simulink model "control_model_1D_v2"  (R2025b)
settings: Solver=VariableStepAuto  StartTime=0.0  StopTime=10  RelTol=1e-3
undefined symbols (not defined in the file): engine_gimbal_speed, engine_max_angle, g, gain, initial_position, initial_teta, initial_velocity, Iy, kd, kd_t, kp, kp_t, Kr, Kx, mass, max_thrust, sigma, static_margin
libraries: simulink_extras x4
settings Model: Creator=marti  LastModifiedBy=marti

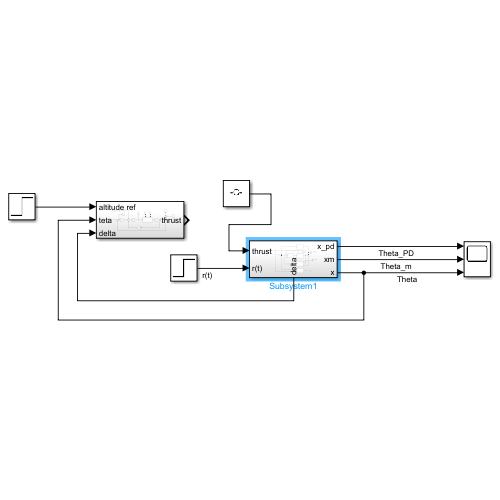
[thumbnail: Simulink's stored preview of the top-level diagram]
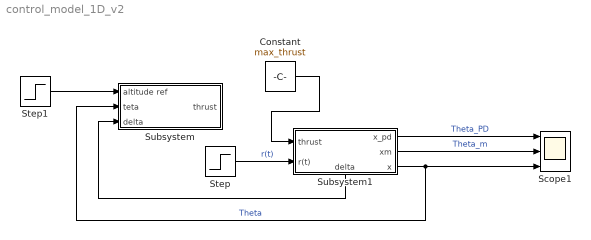
== system control_model_1D_v2 ==
  Constant : Constant  Value=max_thrust
  Scope1 : Scope  NumInputPorts=3
      settings: ActiveDisplayYMinimum=-1.6412064718463906  ActiveDisplayYMaximum=14.77085824661752
  Step : Step  Before=initial_teta  After=10  SampleTime=0
  Step1 : Step  After=30  SampleTime=0
  Subsystem : Subsystem
  Subsystem1 : Subsystem
      settings: PortSchema="{\"entries\":[{\"content\":{\"sides\":[{\"content\":{\"connectorIds\":[\"In1\",\"In2\"]},\"type\":\"ConnectorPlacement.EquallySpacedRectSide\",\"uuid\":\"41c30777-45a1-4158-aee6-2356aa4b2cc5\"},{\"content\":{\"connectorIds\":[\"Out1\",\"Out2\",\"Out3\"],\"side\":\"RIGHT\"},\"type\":\"ConnectorPlacement.EquallySpacedRectSide\",\"uuid\":\"fbc810ba-f647-48d5-9a79-9c3fa84944c8\"},{\"content\":{\"side\":\"TOP\"},\"type\":\"ConnectorPlacement.EquallySpacedRectSide\",\"uuid\":\"5da60fab-04d4-4aae-8ae1-a9a5fc9cdb5d\"},{\"content\":{\"connectorIds\":[\"Out4\"],\"side\":\"BOTTOM\"},\"type\":\"ConnectorPlacement.EquallySpacedRectSide\",\"uuid\":\"fa96aa9e-dc15-4c7b-bdde-b0db6a17889e\"}]},\"type\":\"ConnectorPlacement.EquallySpacedConnector\",\"uuid\":\"2ab61ab6-63dc-40be-af51-040989328b07\"}],\"packageUris\":[\"http://schema.mathworks.com/mf0/Connector/R2020b\"],\"version\":\"1.0\"}"
  wires:
  Step1/1 -> Subsystem/1(altitude ref)
  Step/1 -> Subsystem1/2(r(t))  "r(t)"
  Subsystem1/3(x) -> Subsystem/2(teta), Scope1/3  "Theta"
  Subsystem1/4(delta) -> Subsystem/3(delta)
  Constant/1 -> Subsystem1/1(thrust)
  Subsystem1/2(xm) -> Scope1/2  "Theta_m"
  Subsystem1/1(x_pd) -> Scope1/1  "Theta_PD"

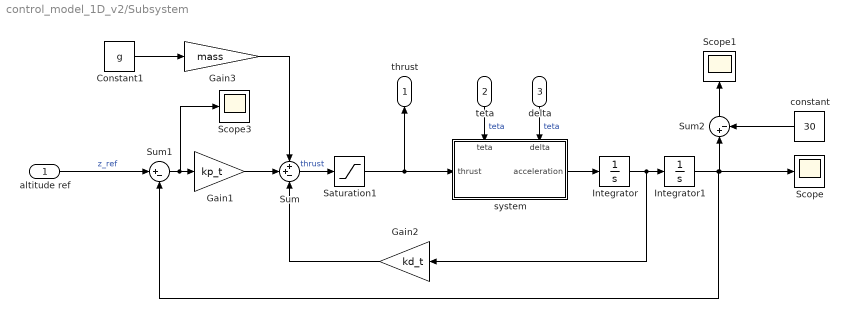
== system control_model_1D_v2/Subsystem ==
  altitude ref : Inport
  teta : Inport  Port=2
  delta : Inport  Port=3
  Constant1 : Constant  Value=g
  Gain1 : Gain  Gain=kp_t
  Gain2 : Gain  Gain=kd_t
  Gain3 : Gain  Gain=mass
  Integrator : Integrator  InitialCondition=initial_velocity
  Integrator1 : Integrator  InitialCondition=initial_position
  Saturation1 : Saturate  UpperLimit=max_thrust  LowerLimit=0
  Scope : Scope
      settings: ActiveDisplayYMinimum=-203.34625268465874  ActiveDisplayYMaximum=578.14958363162873  DataLoggingVariableName=ScopeData7
  Scope1 : Scope
      settings: ActiveDisplayYMinimum=-0.900366360338765  ActiveDisplayYMaximum=1.8353888602601565  DataLoggingVariableName=ScopeData9
  Scope3 : Scope
      settings: ActiveDisplayYMinimum=-1  ActiveDisplayYMaximum=1  DataLoggingVariableName=ScopeData10
  Sum : Sum  Inputs=++-
  Sum1 : Sum  Inputs=|+-
  Sum2 : Sum  Inputs=|+-
  constant : Constant  Value=30
  system : Subsystem
      settings: PortSchema="{\"entries\":[{\"content\":{\"sides\":[{\"content\":{\"connectorIds\":[\"In1\"]},\"type\":\"ConnectorPlacement.EquallySpacedRectSide\",\"uuid\":\"38ff2807-5c3f-4880-9c07-8b6447135695\"},{\"content\":{\"connectorIds\":[\"Out1\"],\"side\":\"RIGHT\"},\"type\":\"ConnectorPlacement.EquallySpacedRectSide\",\"uuid\":\"bc1e5b06-9245-4ba5-abe1-979ca83ec99f\"},{\"content\":{\"connectorIds\":[\"In2\",\"In3\"],\"side\":\"TOP\"},\"type\":\"ConnectorPlacement.EquallySpacedRectSide\",\"uuid\":\"205a83f4-1465-412a-8e3f-6475f5e18be2\"}]},\"type\":\"ConnectorPlacement.EquallySpacedConnector\",\"uuid\":\"dff9f67b-b046-4801-81e2-6dc88e83eb4a\"}],\"packageUris\":[\"http://schema.mathworks.com/mf0/Connector/R2020b\"],\"version\":\"1.0\"}"
  thrust : Outport
  wires:
  system/1(acceleration) -> Integrator/1
  Integrator1/1 -> Scope/1, Sum2/1, Sum1/2
  Gain1/1 -> Sum/2
  Gain2/1 -> Sum/3
  Sum/1 -> Saturation1/1  "thrust"
  Sum1/1 -> Scope3/1, Gain1/1
  Integrator/1 -> Gain2/1, Integrator1/1
  Gain3/1 -> Sum/1
  Constant1/1 -> Gain3/1
  Saturation1/1 -> system/1(thrust), thrust/1
  altitude ref/1 -> Sum1/1  "z_ref"
  teta/1 -> system/2(teta)  "teta"
  constant/1 -> Sum2/2
  Sum2/1 -> Scope1/1
  delta/1 -> system/3(delta)  "teta"

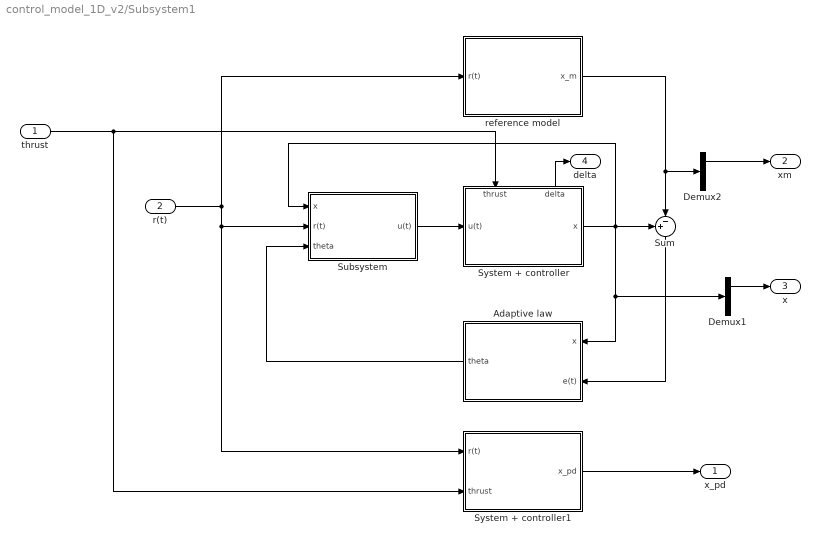
== system control_model_1D_v2/Subsystem1 ==
  thrust : Inport
  r(t) : Inport  Port=2
  Adaptive law : Subsystem  TreatAsAtomicUnit=on
  Demux1 : Demux  Outputs=2
  Demux2 : Demux  Outputs=2
  Subsystem : Subsystem
  Sum : Sum  Inputs=+-|
  System + controller : Subsystem  TreatAsAtomicUnit=on
      settings: PortSchema="{\"entries\":[{\"content\":{\"sides\":[{\"content\":{\"connectorIds\":[\"In1\"]},\"type\":\"ConnectorPlacement.EquallySpacedRectSide\",\"uuid\":\"2888ac6a-c40c-4cbc-ab95-9cb0d58d2b5f\"},{\"content\":{\"connectorIds\":[\"Out1\"],\"side\":\"RIGHT\"},\"type\":\"ConnectorPlacement.EquallySpacedRectSide\",\"uuid\":\"92af2965-0673-45a9-9c50-ea344a811226\"},{\"content\":{\"connectorIds\":[\"In2\",\"Out2\"],\"side\":\"TOP\"},\"type\":\"ConnectorPlacement.EquallySpacedRectSide\",\"uuid\":\"493763d9-5d0c-4185-aada-33137c4c3c69\"}]},\"type\":\"ConnectorPlacement.EquallySpacedConnector\",\"uuid\":\"efbf835c-12ee-4cd9-bf50-b22f4e1c27f3\"}],\"packageUris\":[\"http://schema.mathworks.com/mf0/Connector/R2020b\"],\"version\":\"1.0\"}"
  System + controller1 : Subsystem  TreatAsAtomicUnit=on
  reference model : Subsystem  TreatAsAtomicUnit=on
  x_pd : Outport
  xm : Outport  Port=2
  x : Outport  Port=3
  delta : Outport  Port=4
  wires:
  thrust/1 -> System + controller/2(thrust), System + controller1/2(thrust)
  reference model/1(x_m) -> Demux2/1, Sum/2
  System + controller/1(x) -> Demux1/1, Adaptive law/1(x), Subsystem/1(x), Sum/1
  r(t)/1 -> Subsystem/2(r(t)), System + controller1/1(r(t)), reference model/1(r(t))
  Adaptive law/1(theta) -> Subsystem/3(theta)
  Sum/1 -> Adaptive law/2(e(t))
  System + controller/2(delta) -> delta/1
  System + controller1/1(x_pd) -> x_pd/1
  Demux1/1 -> x/1
  Demux2/1 -> xm/1
  Subsystem/1(u(t)) -> System + controller/1(u(t))

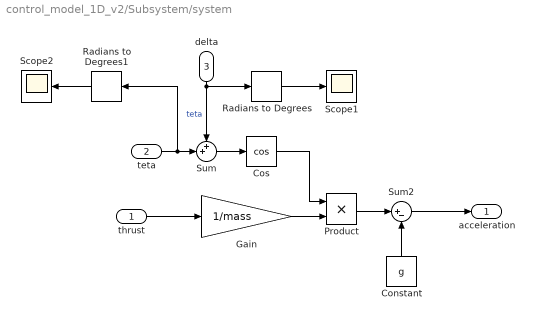
== system control_model_1D_v2/Subsystem/system ==
  thrust : Inport
  teta : Inport  Port=2
  delta : Inport  Port=3
  Constant : Constant  Value=g
  Cos : Trigonometry  Operator=cos
  Gain : Gain  Gain=1/mass
  Product : Product
  Radians to Degrees : simulink_extras/Transformations/Radians to Degrees
  Radians to Degrees1 : simulink_extras/Transformations/Radians to Degrees
  Scope1 : Scope
      settings: ActiveDisplayYMinimum=-1  ActiveDisplayYMaximum=1  DataLoggingVariableName=ScopeData12
  Scope2 : Scope
      settings: ActiveDisplayYMinimum=-1  ActiveDisplayYMaximum=1  DataLoggingVariableName=ScopeData13
  Sum : Sum  Inputs=++|
  Sum2 : Sum  Inputs=|+-
  acceleration : Outport
  wires:
  Constant/1 -> Sum2/2
  Sum2/1 -> acceleration/1
  thrust/1 -> Gain/1
  Gain/1 -> Product/2
  Product/1 -> Sum2/1
  Cos/1 -> Product/1
  teta/1 -> Radians to Degrees1/1, Sum/2
  delta/1 -> Sum/1, Radians to Degrees/1  "teta"
  Sum/1 -> Cos/1
  Radians to Degrees/1 -> Scope1/1
  Radians to Degrees1/1 -> Scope2/1

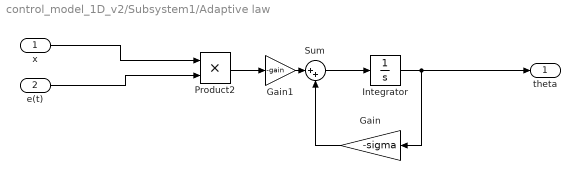
== system control_model_1D_v2/Subsystem1/Adaptive law ==
  x : Inport
  e(t) : Inport  Port=2
  Gain : Gain  Gain=-sigma
  Gain1 : Gain  Gain=-gain
  Integrator : Integrator
  Product2 : Product
  Sum : Sum  Inputs=|++
  theta : Outport
  wires:
  Integrator/1 -> Gain/1, theta/1
  Sum/1 -> Integrator/1
  Gain/1 -> Sum/2
  Gain1/1 -> Sum/1
  Product2/1 -> Gain1/1
  x/1 -> Product2/1
  e(t)/1 -> Product2/2

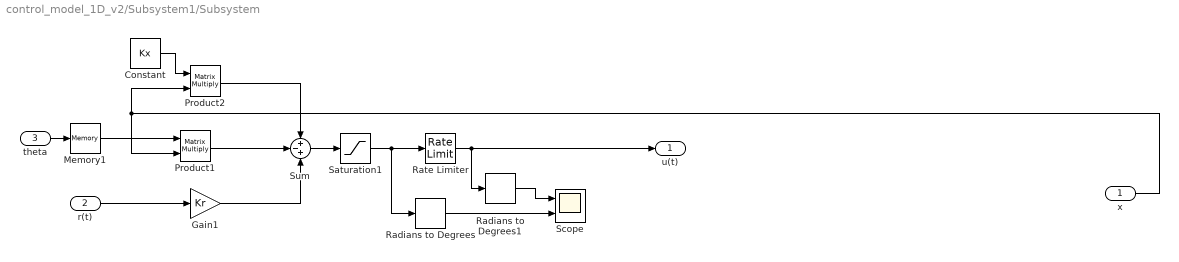
== system control_model_1D_v2/Subsystem1/Subsystem ==
  x : Inport
  r(t) : Inport  Port=2
  theta : Inport  Port=3
  Constant : Constant  Value=Kx  VectorParams1D=off
  Gain1 : Gain  Gain=Kr
  Memory1 : Memory
  Product1 : Product  Multiplication=Matrix(*)
  Product2 : Product  Multiplication=Matrix(*)
  Radians to Degrees : simulink_extras/Transformations/Radians to Degrees
  Radians to Degrees1 : simulink_extras/Transformations/Radians to Degrees
  Rate Limiter : RateLimiter  RisingSlewLimit=engine_gimbal_speed  FallingSlewLimit=-engine_gimbal_speed  SampleTimeMode=inherited
  Saturation1 : Saturate  UpperLimit=engine_max_angle  LowerLimit=-engine_max_angle
  Scope : Scope  NumInputPorts=2
      settings: ActiveDisplayYMinimum=-0.14117420065901104  ActiveDisplayYMaximum=0.22600812143216731
  Sum : Sum  Inputs=+-+
  u(t) : Outport
  wires:
  Radians to Degrees1/1 -> Scope/1
  Memory1/1 -> Product1/1
  r(t)/1 -> Gain1/1
  x/1 -> Product2/2, Product1/2
  Product2/1 -> Sum/1
  Saturation1/1 -> Radians to Degrees/1, Rate Limiter/1
  theta/1 -> Memory1/1
  Constant/1 -> Product2/1
  Gain1/1 -> Sum/3
  Rate Limiter/1 -> u(t)/1, Radians to Degrees1/1
  Radians to Degrees/1 -> Scope/2
  Sum/1 -> Saturation1/1
  Product1/1 -> Sum/2

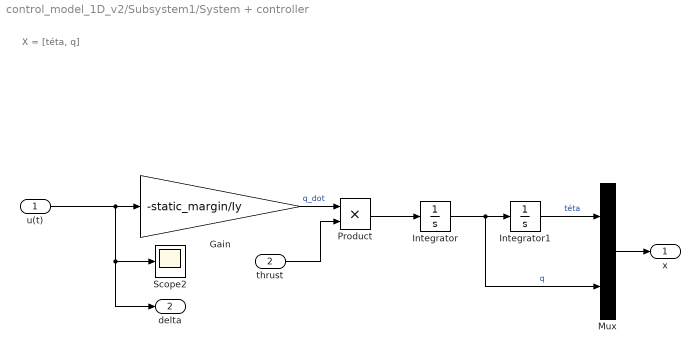
== system control_model_1D_v2/Subsystem1/System + controller ==
  note: X = [téta, q]
  u(t) : Inport
  thrust : Inport  Port=2
  Gain : Gain  Gain=-static_margin/Iy
  Integrator : Integrator
  Integrator1 : Integrator  InitialCondition=initial_teta
  Mux : Mux  Inputs=2
  Product : Product
  Scope2 : Scope
      settings: ActiveDisplayYMinimum=-1  ActiveDisplayYMaximum=1  DataLoggingVariableName=ScopeData3
  x : Outport
  delta : Outport  Port=2
  wires:
  Integrator/1 -> Mux/2, Integrator1/1  "q"
  Gain/1 -> Product/1  "q_dot"
  Product/1 -> Integrator/1
  thrust/1 -> Product/2
  Integrator1/1 -> Mux/1  "téta"
  Mux/1 -> x/1
  u(t)/1 -> delta/1, Scope2/1, Gain/1

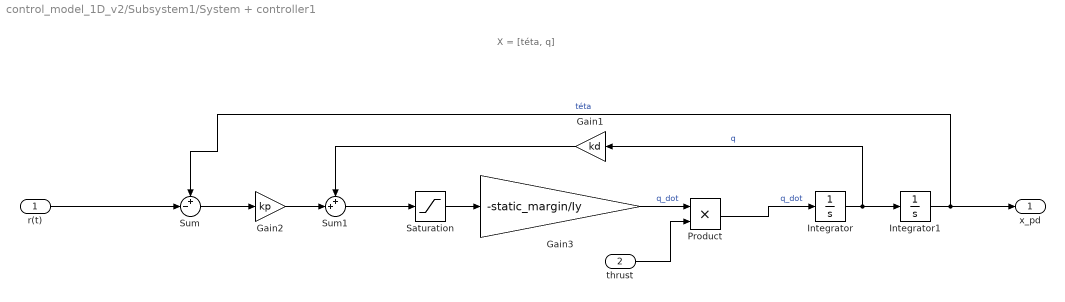
== system control_model_1D_v2/Subsystem1/System + controller1 ==
  note: X = [téta, q]
  r(t) : Inport
  thrust : Inport  Port=2
  Gain1 : Gain  Gain=kd
  Gain2 : Gain  Gain=kp
  Gain3 : Gain  Gain=-static_margin/Iy
  Integrator : Integrator
  Integrator1 : Integrator  InitialCondition=initial_teta
  Product : Product
  Saturation : Saturate  UpperLimit=engine_max_angle  LowerLimit=-engine_max_angle
  Sum : Sum  Inputs=+-|
  Sum1 : Sum  Inputs=++|
  x_pd : Outport
  wires:
  Product/1 -> Integrator/1  "q_dot"
  Integrator/1 -> Gain1/1, Integrator1/1  "q"
  Integrator1/1 -> Sum/1, x_pd/1  "téta"
  Sum/1 -> Gain2/1
  r(t)/1 -> Sum/2
  Sum1/1 -> Saturation/1
  Gain1/1 -> Sum1/1
  Gain2/1 -> Sum1/2
  thrust/1 -> Product/2
  Gain3/1 -> Product/1  "q_dot"
  Saturation/1 -> Gain3/1

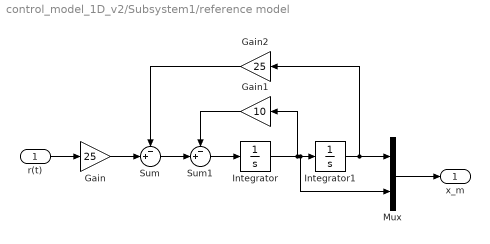
== system control_model_1D_v2/Subsystem1/reference model ==
  r(t) : Inport
  Gain : Gain  Gain=25
  Gain1 : Gain  Gain=10
  Gain2 : Gain  Gain=25
  Integrator : Integrator
  Integrator1 : Integrator
  Mux : Mux  Inputs=2
  Sum : Sum  Inputs=-+|
  Sum1 : Sum  Inputs=-+|
  x_m : Outport
  wires:
  r(t)/1 -> Gain/1
  Integrator/1 -> Gain1/1, Mux/2, Integrator1/1
  Sum/1 -> Sum1/2
  Sum1/1 -> Integrator/1
  Integrator1/1 -> Gain2/1, Mux/1
  Gain/1 -> Sum/2
  Gain2/1 -> Sum/1
  Gain1/1 -> Sum1/1
  Mux/1 -> x_m/1
